simulink model "model_sin_actuator"  (R2015b)
settings: Solver=VariableStepAuto  StartTime=0.0  StopTime=10.0  RelTol=1e-3
libraries: fuzblock x1
settings Model: Creator=metalhead  LastModifiedBy=metalhead

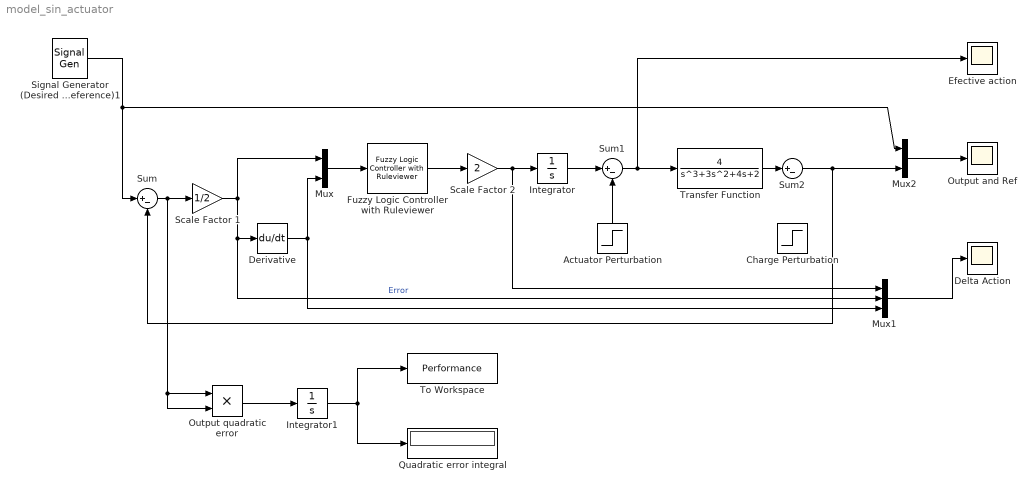
== system model_sin_actuator ==
  Actuator Perturbation : Step  Time=200  After=0.1  SampleTime=0
  "Charge Perturbation " : Step  Time=200  After=0.1  SampleTime=0
  Delta Action : Scope
  Derivative : Derivative
  Efective action : Scope
  Fuzzy Logic Controller with Ruleviewer : fuzblock/Fuzzy Logic  Controller  with Ruleviewer  fismatrix=controller  Ts=2
  Integrator : Integrator
  Integrator1 : Integrator
  Mux : Mux  Inputs=2
  Mux1 : Mux  Inputs=3
  Mux2 : Mux  Inputs=2
  Output and Ref : Scope
  Output quadratic error : Product  RndMeth=Zero
  Quadratic error integral : Display
  Scale Factor 1 : Gain  Gain=1/2
  Scale Factor 2 : Gain  Gain=2
  Signal Generator (Desired Reference)1 : SignalGenerator  Amplitude=-1  Frequency=0.01  Units=rad/sec
  Sum : Sum  Inputs=|+-
  Sum1 : Sum  Inputs=|+-
  Sum2 : Sum  Inputs=|+-
  To Workspace : ToWorkspace  VariableName=Performance  SaveFormat=Structure  SampleTime=-1
  Transfer Function : TransferFcn  Numerator=[4]  Denominator=[1 3 4 2]
  wires:
  Signal Generator (Desired Reference)1/1 -> Sum/1, Mux2/1
  Sum/1 -> Scale Factor 1/1, Output quadratic error/1, Output quadratic error/2
  Scale Factor 1/1 -> Mux/1, Derivative/1, Mux1/2  "Error"
  Derivative/1 -> Mux/2, Mux1/3
  Mux1/1 -> Delta Action/1
  Mux/1 -> Fuzzy Logic Controller with Ruleviewer/1
  Fuzzy Logic Controller with Ruleviewer/1 -> Scale Factor 2/1
  Scale Factor 2/1 -> Integrator/1, Mux1/1
  Integrator/1 -> Sum1/1
  Sum1/1 -> Efective action/1, Transfer Function/1
  Sum2/1 -> Mux2/2, Sum/2
  Mux2/1 -> Output and Ref/1
  Output quadratic error/1 -> Integrator1/1
  Integrator1/1 -> Quadratic error integral/1, To Workspace/1
  Transfer Function/1 -> Sum2/1
  Actuator Perturbation/1 -> Sum1/2
